simulink model "nad_send"  (R2017b)
settings: Solver=VariableStepAuto  StartTime=0.0  StopTime=10  RelTol=1e-3
libraries: lib_ed247 x1
settings Model: Creator=odufour  LastModifiedBy=odufour
settings DataIOCC: ExternalInput=nadtestinputdataset  LoadExternalInput=on  SignalLoggingName=nadtestinputdataset
settings CodeAppCC: StateflowObjectComments=on

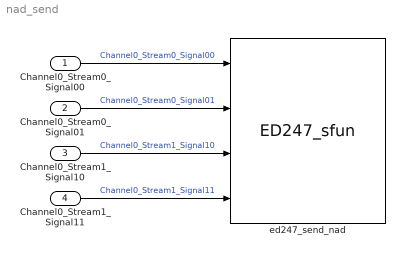
== system nad_send ==
  Channel0_Stream0_Signal00 : Inport  SampleTime=1  Interpolate=off
  Channel0_Stream0_Signal01 : Inport  Port=2  SampleTime=1  Interpolate=off
  Channel0_Stream1_Signal10 : Inport  Port=3  SampleTime=1  Interpolate=off
  Channel0_Stream1_Signal11 : Inport  Port=4  SampleTime=1  Interpolate=off
  ed247_send_nad : lib_ed247/ED247_sfun  configurationFilename='nad_mc_1.xml'  enableLog=off  logFilename=''
      settings: SourceProductName=Airbus ED247
  wires:
  Channel0_Stream0_Signal00/1 -> ed247_send_nad/1  "Channel0_Stream0_Signal00"
  Channel0_Stream0_Signal01/1 -> ed247_send_nad/2  "Channel0_Stream0_Signal01"
  Channel0_Stream1_Signal10/1 -> ed247_send_nad/3  "Channel0_Stream1_Signal10"
  Channel0_Stream1_Signal11/1 -> ed247_send_nad/4  "Channel0_Stream1_Signal11"
